simulink model "betavars"  (Simulink 7.6)
settings: Solver=ode15s  StartTime=0  StopTime=100  RelTol=1e-4  AbsTol=1e-5
values from neighbouring files (symbols this model uses):
  alphaC = p(16)    [betasim.m]    (also in betasim_IE.m)
  alphaP = p(13)    [betasim.m]    (also in betasim_IE.m)
  Ca0 = fCa(p,paux.c(1,1))    [betasim.m]    (also in betasim_IE.m)
  CaGlu0 = fCaGlu(p,paux.c(1,1),paux.g(1,1))    [betasim.m]    (also in betasim_IE.m)
  delayC = p(15)    [betasim.m]    (also in betasim_IE.m)
  delayP = p(14)    [betasim.m]    (also in betasim_IE.m)
settings Model: Creator=Valentina  LastModifiedBy=Andrea Mari
settings DataIOCC: SaveOutput=off  SignalLogging=off  SaveTime=off
settings OptimizationCC: InitFltsAndDblsToZero=on
settings DebuggingCC: SaveWithParameterizedLinksMsg=none  SignalResolutionControl=TryResolveAllWithWarning  SolverPrmCheckMsg=none  MultiTaskCondExecSysMsg=none  StrictBusMsg=Warning
settings RTWCC: IncludeERTFirstTime=on
settings GRTTargetCC: TargetFcnLib=ansi_tfl_tmw.mat

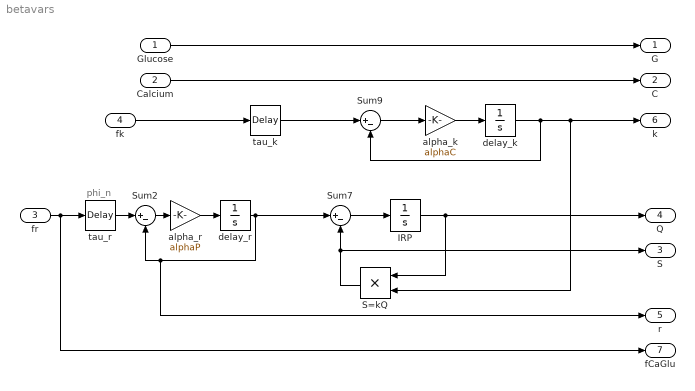
== system betavars ==
  note: phi_n
  Glucose : Inport
  Calcium : Inport  Port=2
  fr : Inport  Port=3
  fk : Inport  Port=4
  IRP : Integrator  InitialCondition=CaGlu0/Ca0
  S=kQ : Product  RndMeth=Zero
  Sum2 : Sum  Inputs=|+-  SaturateOnIntegerOverflow=on
  Sum7 : Sum  Inputs=|+-
  Sum9 : Sum  Inputs=|+-
  alpha_k : Gain  Gain=alphaC
  alpha_r : Gain  Gain=alphaP  SaturateOnIntegerOverflow=on  OutDataTypeStr=Inherit: Same as input  ParamDataTypeStr=Inherit: Same as input
  delay_k : Integrator  InitialCondition=Ca0
  delay_r : Integrator  InitialCondition=CaGlu0
  tau_k : TransportDelay  DelayTime=delayC  InitialOutput=Ca0
  tau_r : TransportDelay  DelayTime=delayP  InitialOutput=CaGlu0
  G : Outport
  C : Outport  Port=2
  S : Outport  Port=3
  Q : Outport  Port=4
  r : Outport  Port=5
  k : Outport  Port=6
  fCaGlu : Outport  Port=7
  wires:
  delay_r/1 -> Sum7/1, Sum2/2, r/1
  Sum2/1 -> alpha_r/1
  tau_r/1 -> Sum2/1
  alpha_r/1 -> delay_r/1
  delay_k/1 -> S=kQ/2, k/1, Sum9/2
  Sum7/1 -> IRP/1
  IRP/1 -> S=kQ/1, Q/1
  alpha_k/1 -> delay_k/1
  Sum9/1 -> alpha_k/1
  S=kQ/1 -> Sum7/2, S/1
  tau_k/1 -> Sum9/1
  Glucose/1 -> G/1
  Calcium/1 -> C/1
  fr/1 -> fCaGlu/1, tau_r/1
  fk/1 -> tau_k/1
